simulink model "gm_HDL_pfc_gold_fi_og"  (R2024b)
settings: Solver=FixedStepDiscrete  StartTime=0.0  StopTime=.2  RelTol=1e-3
InitFcn:
  | fidelity_pfc_vals;
  | nbits=(2^12)-2;
  | A_mat = fi(stateSpaceParameters_1.Ad,1,25,24);
  | B_mat = fi(stateSpaceParameters_1.Bd,1,25,31);
  | C_mat = fi(stateSpaceParameters_1.Cd,1,25,20);
  | D_mat = fi(stateSpaceParameters_1.Dd,1,25,19);
  | X0_mat= fi(stateSpaceParameters_1.X0,1,25,14);
  | load('C:\Users\Angel\Desktop\hil\pfc3ph\matlab\sim\sschdl\pfc_desktop\stateSpaceParameters.mat');
undefined symbols (not defined in the file or in its folder): a, b, c, fsw, t_ss, tsw
libraries: simulink x39, hdlmdlgenlib x24, hdlsllib x9, mcbcontrolslib x5, dspsrcs4 x3, slpidlib x2, spsSVPWMGenerator2LevelLib x1, spsPLL3phLib x1, fillib x1
(part 1 of 4)
settings Model: Creator=angro  LastModifiedBy=Angel
settings OptimizationCC: BlockReduction=off  ConditionallyExecuteInputs=off  DefaultParameterBehavior=Inlined  InheritOutputTypeSmallerThanSingle=on  DefaultUnderspecifiedDataType=single
settings DebuggingCC: SignalRangeChecking=warning  AlgebraicLoopMsg=none  ArtificialAlgebraicLoopMsg=error  InheritedTsInSrcMsg=none  SingleTaskRateTransMsg=error  UnconnectedInputMsg=warning  UnconnectedOutputMsg=warning  UnconnectedLineMsg=warning
settings HardwareCC: ProdBitPerPointer=32  ProdBitPerSizeT=32  ProdBitPerPtrDiffT=32  ProdLargestAtomicFloat=None  ProdIntDivRoundTo=Undefined  ProdEndianess=Unspecified  ProdWordSize=32  ProdHWDeviceType=ASIC/FPGA->ASIC/FPGA  TargetBitPerPointer=64  TargetBitPerSizeT=64  TargetBitPerPtrDiffT=64  TargetLongLongMode=on  TargetIntDivRoundTo=Zero  TargetEndianess=LittleEndian  TargetWordSize=64  TargetHWDeviceType=Custom Processor->MATLAB Host Computer  ProdEqTarget=off

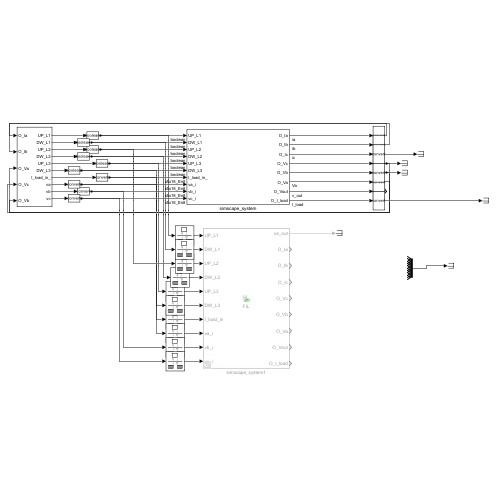
[thumbnail: Simulink's stored preview of the top-level diagram]
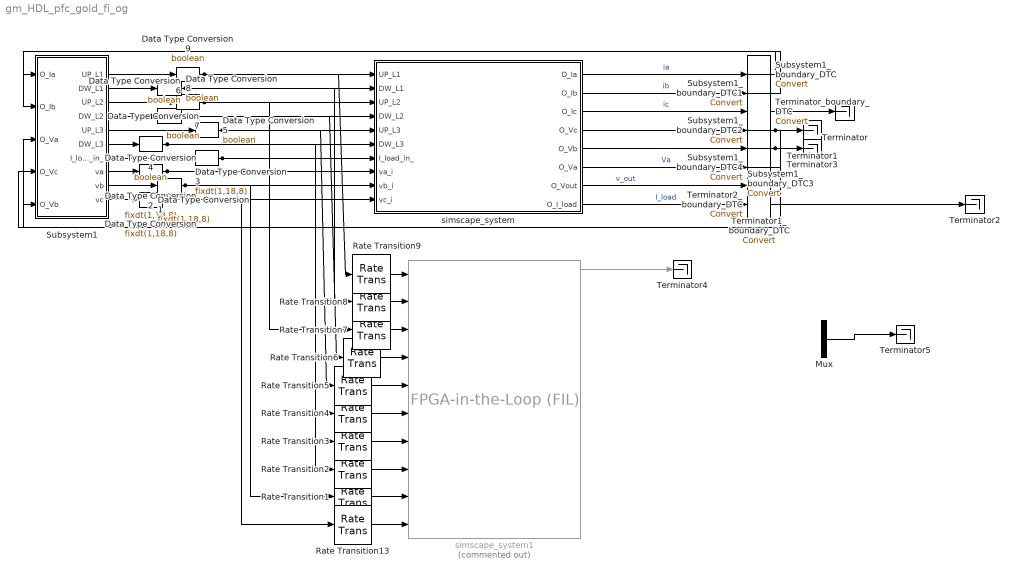
== system gm_HDL_pfc_gold_fi_og ==
  Data Type Conversion{,1..3} (4 alike) : DataTypeConversion  OutDataTypeStr=fixdt(1,18,8)  SaturateOnIntegerOverflow=off  RndMeth=Floor
  Data Type Conversion{4..9} (6 alike) : DataTypeConversion  OutDataTypeStr=boolean  SaturateOnIntegerOverflow=off  RndMeth=Floor
  Mux : Mux  Inputs=9
  Rate Transition{1..9,13} (10 alike) : RateTransition
  Subsystem1 : Subsystem
  Subsystem1_boundary_DTC{,1..4} (5 alike) : DataTypeConversion
  Terminator{,1..5} (6 alike) : Terminator
  Terminator1_boundary_DTC : DataTypeConversion
  Terminator2_boundary_DTC : DataTypeConversion
  Terminator_boundary_DTC : DataTypeConversion
  simscape_system : Subsystem
  simscape_system1 : fillib/FPGA-in-the-Loop (FIL)  Commented=on  ForceInterfaceUpdate=0.63368
  wires:
  simscape_system/8(O_I_load) -> Terminator2_boundary_DTC/1  "I_load"
  simscape_system/7(O_Vout) -> Terminator1_boundary_DTC/1  "v_out"
  simscape_system/6(O_Va) -> Subsystem1_boundary_DTC4/1  "Va"
  simscape_system/5(O_Vb) -> Subsystem1_boundary_DTC3/1
  simscape_system/4(O_Vc) -> Subsystem1_boundary_DTC2/1
  simscape_system/3(O_Ic) -> Terminator_boundary_DTC/1  "ic"
  simscape_system/2(O_Ib) -> Subsystem1_boundary_DTC1/1  "ib"
  simscape_system/1(O_Ia) -> Subsystem1_boundary_DTC/1  "ia"
  Mux/1 -> Terminator5/1
  Rate Transition9/1 -> simscape_system1/1
  Rate Transition8/1 -> simscape_system1/2
  Rate Transition7/1 -> simscape_system1/3
  Rate Transition6/1 -> simscape_system1/4
  Rate Transition5/1 -> simscape_system1/5
  Rate Transition4/1 -> simscape_system1/6
  Rate Transition3/1 -> simscape_system1/7
  Rate Transition2/1 -> simscape_system1/8
  Rate Transition1/1 -> simscape_system1/9
  Rate Transition13/1 -> simscape_system1/10
  simscape_system1/1 -> Terminator4/1
  Subsystem1_boundary_DTC4/1 -> Subsystem1/3(O_Va)
  Subsystem1_boundary_DTC3/1 -> Subsystem1/5(O_Vb), Terminator3/1
  Subsystem1_boundary_DTC2/1 -> Subsystem1/4(O_Vc), Terminator1/1
  Subsystem1_boundary_DTC1/1 -> Subsystem1/2(O_Ib)
  Subsystem1_boundary_DTC/1 -> Subsystem1/1(O_Ia)
  Terminator2_boundary_DTC/1 -> Terminator2/1
  Terminator_boundary_DTC/1 -> Terminator/1
  Data Type Conversion9/1 -> Rate Transition9/1, simscape_system/1(UP_L1)
  Data Type Conversion8/1 -> Rate Transition8/1, simscape_system/2(DW_L1)
  Data Type Conversion7/1 -> simscape_system/3(UP_L2), Rate Transition7/1
  Data Type Conversion6/1 -> Rate Transition6/1, simscape_system/4(DW_L2)
  Data Type Conversion5/1 -> Rate Transition5/1, simscape_system/5(UP_L3)
  Data Type Conversion4/1 -> Rate Transition4/1, simscape_system/6(DW_L3)
  Data Type Conversion3/1 -> Rate Transition3/1, simscape_system/7(I_load_in_)
  Data Type Conversion2/1 -> Rate Transition2/1, simscape_system/8(va_i)
  Data Type Conversion1/1 -> simscape_system/9(vb_i), Rate Transition1/1
  Data Type Conversion/1 -> simscape_system/10(vc_i), Rate Transition13/1
  Subsystem1/10(vc) -> Data Type Conversion/1
  Subsystem1/9(vb) -> Data Type Conversion1/1
  Subsystem1/8(va) -> Data Type Conversion2/1
  Subsystem1/6(DW_L3) -> Data Type Conversion4/1
  Subsystem1/5(UP_L3) -> Data Type Conversion5/1
  Subsystem1/4(DW_L2) -> Data Type Conversion6/1
  Subsystem1/3(UP_L2) -> Data Type Conversion7/1
  Subsystem1/2(DW_L1) -> Data Type Conversion8/1
  Subsystem1/1(UP_L1) -> Data Type Conversion9/1
  Subsystem1/7(I_load_in_) -> Data Type Conversion3/1

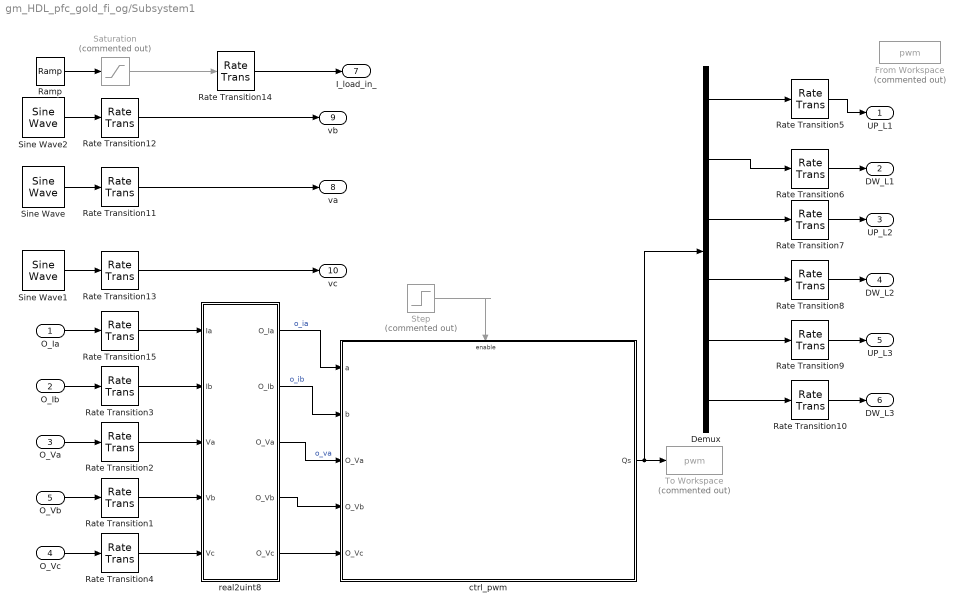
== system gm_HDL_pfc_gold_fi_og/Subsystem1 ==
  O_Ia : Inport
  O_Ib : Inport  Port=2
  O_Va : Inport  Port=3
  O_Vc : Inport  Port=4
  O_Vb : Inport  Port=5
  Demux : Demux  Outputs=6
  From Workspace : FromWorkspace  Commented=on  VariableName=pwm  SampleTime=t_ss  Interpolate=off  ZeroCross=off  OutputAfterFinalValue=Holding final value
  Ramp : simulink/Sources/Ramp  slope=1/50  start=2/50  InitialOutput=0
  Rate Transition{1..13,15} (14 alike) : RateTransition
  Rate Transition14 : RateTransition  OutPortSampleTime=t_ss
  Saturation : Saturate  Commented=on  UpperLimit=2
  Sine Wave : dspsrcs4/Sine Wave  Amplitude=325  Frequency=50  Phase=0  SampleMode=Discrete  OutComplex=Real  CompMethod=Table lookup  TableSize=Speed  SampleTime=tsw  SamplesPerFrame=1  ResetState=Restart at time zero  OutputFrames=off  dataType=double  wordLen=16  udDataType=sfix(16)  fracBitsMode=Best precision  numFracBits=15  OutDataTypeStr=double  LastOutDataTypeStr=double
  Sine Wave1 : dspsrcs4/Sine Wave  Amplitude=325  Frequency=50  Phase=2*pi/3  SampleMode=Discrete  OutComplex=Real  CompMethod=Table lookup  TableSize=Speed  SampleTime=tsw  SamplesPerFrame=1  ResetState=Restart at time zero  OutputFrames=off  dataType=double  wordLen=16  udDataType=sfix(16)  fracBitsMode=Best precision  numFracBits=15  OutDataTypeStr=double  LastOutDataTypeStr=double
  Sine Wave2 : dspsrcs4/Sine Wave  Amplitude=325  Frequency=50  Phase=-2*pi/3  SampleMode=Discrete  OutComplex=Real  CompMethod=Table lookup  TableSize=Speed  SampleTime=tsw  SamplesPerFrame=1  ResetState=Restart at time zero  OutputFrames=off  dataType=double  wordLen=16  udDataType=sfix(16)  fracBitsMode=Best precision  numFracBits=15  OutDataTypeStr=double  LastOutDataTypeStr=double
  Step : Step  Commented=on  Time=2/50  SampleTime=0
  To Workspace : ToWorkspace  Commented=on  VariableName=pwm  SaveFormat=Timeseries  SampleTime=-1
  ctrl_pwm : Subsystem
  real2uint8 : Subsystem
  UP_L1 : Outport
  DW_L1 : Outport  Port=2
  UP_L2 : Outport  Port=3
  DW_L2 : Outport  Port=4
  UP_L3 : Outport  Port=5
  DW_L3 : Outport  Port=6
  I_load_in_ : Outport  Port=7
  va : Outport  Port=8
  vb : Outport  Port=9
  vc : Outport  Port=10
  wires:
  Rate Transition9/1 -> UP_L3/1
  Rate Transition7/1 -> UP_L2/1
  Rate Transition6/1 -> DW_L1/1
  Rate Transition5/1 -> UP_L1/1
  Demux/4 -> Rate Transition8/1
  Demux/3 -> Rate Transition7/1
  Demux/2 -> Rate Transition6/1
  Demux/6 -> Rate Transition10/1
  Demux/1 -> Rate Transition5/1
  Demux/5 -> Rate Transition9/1
  ctrl_pwm/1(Qs) -> To Workspace/1, Demux/1
  real2uint8/5(O_Vc) -> ctrl_pwm/5(O_Vc)
  real2uint8/3(O_Va) -> ctrl_pwm/3(O_Va)  "o_va"
  real2uint8/2(O_Ib) -> ctrl_pwm/2(b)  "o_ib"
  real2uint8/1(O_Ia) -> ctrl_pwm/1(a)  "o_ia"
  real2uint8/4(O_Vb) -> ctrl_pwm/4(O_Vb)
  Step/1 -> ctrl_pwm/Enable
  Rate Transition14/1 -> I_load_in_/1
  Rate Transition10/1 -> DW_L3/1
  Rate Transition4/1 -> real2uint8/5(Vc)
  Rate Transition13/1 -> vc/1
  Rate Transition1/1 -> real2uint8/4(Vb)
  Rate Transition11/1 -> va/1
  Rate Transition3/1 -> real2uint8/2(Ib)
  Rate Transition12/1 -> vb/1
  Rate Transition2/1 -> real2uint8/3(Va)
  O_Vc/1 -> Rate Transition4/1
  O_Ia/1 -> Rate Transition15/1
  O_Va/1 -> Rate Transition2/1
  O_Vb/1 -> Rate Transition1/1
  O_Ib/1 -> Rate Transition3/1
  Sine Wave/1 -> Rate Transition11/1
  Rate Transition8/1 -> DW_L2/1
  Sine Wave1/1 -> Rate Transition13/1
  Saturation/1 -> Rate Transition14/1
  Sine Wave2/1 -> Rate Transition12/1
  Rate Transition15/1 -> real2uint8/1(Ia)
  Ramp/1 -> Saturation/1

== system gm_HDL_pfc_gold_fi_og/simscape_system ==
  UP_L1 : Inport  OutDataTypeStr=boolean  PortDimensions=1  SampleTime=5.12820512820513e-07
  DW_L1 : Inport  Port=2  OutDataTypeStr=boolean  PortDimensions=1  SampleTime=5.12820512820513e-07
  UP_L2 : Inport  Port=3  OutDataTypeStr=boolean  PortDimensions=1  SampleTime=5.12820512820513e-07
  DW_L2 : Inport  Port=4  OutDataTypeStr=boolean  PortDimensions=1  SampleTime=5.12820512820513e-07
  UP_L3 : Inport  Port=5  OutDataTypeStr=boolean  PortDimensions=1  SampleTime=5.12820512820513e-07
  DW_L3 : Inport  Port=6  OutDataTypeStr=boolean  PortDimensions=1  SampleTime=5.12820512820513e-07
  I_load_in_ : Inport  Port=7  OutDataTypeStr=fixdt(1, 18, 8)  PortDimensions=1  SampleTime=5.12820512820513e-07
  va_i : Inport  Port=8  OutDataTypeStr=fixdt(1, 18, 8)  PortDimensions=1  SampleTime=5.12820512820513e-07  LockScale=on
  vb_i : Inport  Port=9  OutDataTypeStr=fixdt(1, 18, 8)  PortDimensions=1  SampleTime=5.12820512820513e-07  LockScale=on
  vc_i : Inport  Port=10  OutDataTypeStr=fixdt(1, 18, 8)  PortDimensions=1  SampleTime=5.12820512820513e-07  LockScale=on
  simscape_system : Subsystem
  t{,1..7} (8 alike) : RateTransition  InitialCondition=double(0)  OutPortSampleTimeOpt=Multiple of input port sample time  OutPortSampleTimeMultiple=49
  O_Ia : Outport  SampleTime=5.12820512820513e-07
  O_Ib : Outport  Port=2  SampleTime=5.12820512820513e-07
  O_Ic : Outport  Port=3  SampleTime=5.12820512820513e-07
  O_Vc : Outport  Port=4  SampleTime=5.12820512820513e-07
  O_Vb : Outport  Port=5  SampleTime=5.12820512820513e-07
  O_Va : Outport  Port=6  SampleTime=5.12820512820513e-07
  O_Vout : Outport  Port=7  SampleTime=5.12820512820513e-07
  O_I_load : Outport  Port=8  SampleTime=5.12820512820513e-07
  wires:
  UP_L1/1 -> simscape_system/1(UP_L1)
  DW_L1/1 -> simscape_system/2(DW_L1)
  UP_L3/1 -> simscape_system/5(UP_L3)
  UP_L2/1 -> simscape_system/3(UP_L2)
  DW_L2/1 -> simscape_system/4(DW_L2)
  I_load_in_/1 -> simscape_system/7(I_load_in_)
  DW_L3/1 -> simscape_system/6(DW_L3)
  va_i/1 -> simscape_system/8(va_i)
  vb_i/1 -> simscape_system/9(vb_i)
  vc_i/1 -> simscape_system/10(vc_i)
  t1/1 -> O_Ic/1
  simscape_system/1(O_Ia) -> t7/1
  simscape_system/2(O_Ib) -> t/1
  simscape_system/3(O_Ic) -> t1/1
  simscape_system/4(O_Vc) -> t2/1
  simscape_system/5(O_Vb) -> t3/1
  simscape_system/6(O_Va) -> t4/1
  t6/1 -> O_I_load/1
  simscape_system/7(O_Vout) -> t5/1
  simscape_system/8(O_I_load) -> t6/1
  t7/1 -> O_Ia/1
  t/1 -> O_Ib/1
  t2/1 -> O_Vc/1
  t3/1 -> O_Vb/1
  t4/1 -> O_Va/1
  t5/1 -> O_Vout/1

== system gm_HDL_pfc_gold_fi_og/Subsystem1/ctrl_pwm ==
  a : Inport
  b : Inport  Port=2
  O_Va : Inport  Port=3
  O_Vb : Inport  Port=4
  O_Vc : Inport  Port=5
  Enable : EnablePort
  PI_CTRL : Subsystem
  SVPWM : Subsystem
  transforms : Subsystem
  Qs : Outport
  wires:
  O_Vb/1 -> transforms/4(In4)
  O_Va/1 -> transforms/3(In3)
  b/1 -> transforms/2(b)
  PI_CTRL/2(Vq_inductor) -> SVPWM/3(Vq_inductor)
  SVPWM/1(P) -> Qs/1  "Qs"
  transforms/2(iq) -> PI_CTRL/2(iq)
  O_Vc/1 -> transforms/5(In5)
  a/1 -> transforms/1(a)
  PI_CTRL/1(Vd_inductor) -> SVPWM/1(Vd_inductor)
  transforms/3(angle) -> SVPWM/2(angle)
  transforms/1(id) -> PI_CTRL/1(id)

== system gm_HDL_pfc_gold_fi_og/Subsystem1/real2uint8 ==
  Ia : Inport
  Ib : Inport  Port=2
  Va : Inport  Port=3
  Vb : Inport  Port=4
  Vc : Inport  Port=5
  Add2 : Sum  Inputs=-+  OutDataTypeStr=Inherit: Same as first input
  Add3 : Sum  Inputs=+-
  Constant : Constant  Value=40  SampleTime=-1
  Constant1 : Constant  Value=420  SampleTime=-1
  Demux : Demux  Outputs=3
  Demux1 : Demux  Outputs=2
  Gain2 : Gain  Gain=80/nbits  OutDataTypeStr=Inherit: Same as input
  Gain5 : Gain  Gain=840/nbits  OutDataTypeStr=Inherit: Same as input
  Mux : Mux  Inputs=3
  Mux1 : Mux  Inputs=2
  O_Ia : Outport
  O_Ib : Outport  Port=2
  O_Va : Outport  Port=3
  O_Vb : Outport  Port=4
  O_Vc : Outport  Port=5
  wires:
  Add3/1 -> Demux/1
  Add2/1 -> Demux1/1
  Gain2/1 -> Add2/2
  Gain5/1 -> Add3/1
  Mux/1 -> Gain5/1
  Mux1/1 -> Gain2/1
  Demux1/2 -> O_Ia/1
  Demux1/1 -> O_Ib/1
  Demux/3 -> O_Va/1
  Demux/2 -> O_Vc/1
  Constant/1 -> Add2/1
  Constant1/1 -> Add3/2
  Demux/1 -> O_Vb/1
  Ib/1 -> Mux1/1
  Vc/1 -> Mux/2
  Ia/1 -> Mux1/2  "rIA"
  Vb/1 -> Mux/1
  Va/1 -> Mux/3

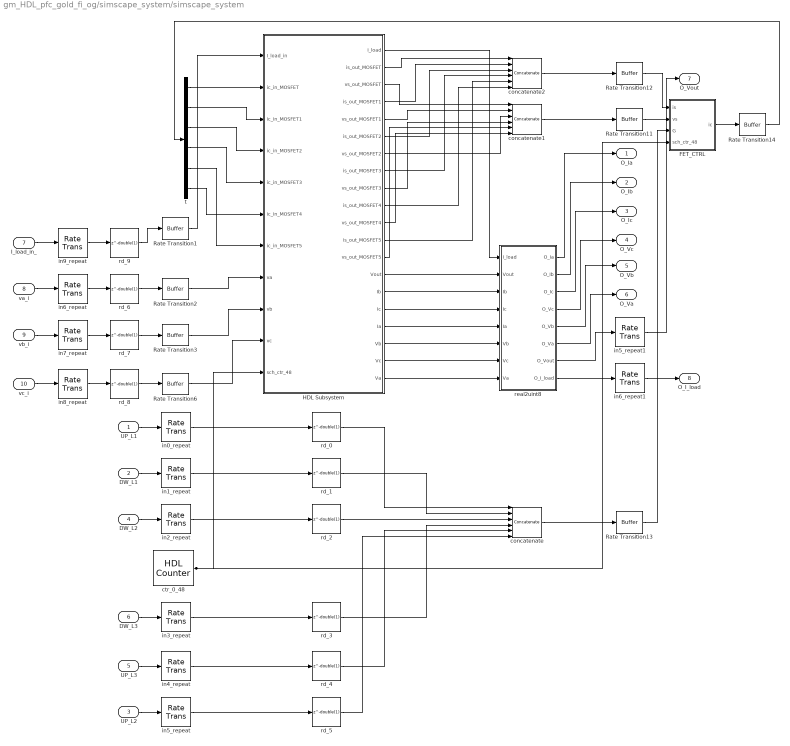
== system gm_HDL_pfc_gold_fi_og/simscape_system/simscape_system ==
  UP_L1 : Inport  OutDataTypeStr=boolean  SampleTime=5.12820512820513e-07
  DW_L1 : Inport  Port=2  OutDataTypeStr=boolean  SampleTime=5.12820512820513e-07
  UP_L2 : Inport  Port=3  OutDataTypeStr=boolean  SampleTime=5.12820512820513e-07
  DW_L2 : Inport  Port=4  OutDataTypeStr=boolean  SampleTime=5.12820512820513e-07
  UP_L3 : Inport  Port=5  OutDataTypeStr=boolean  SampleTime=5.12820512820513e-07
  DW_L3 : Inport  Port=6  OutDataTypeStr=boolean  SampleTime=5.12820512820513e-07
  I_load_in_ : Inport  Port=7  OutDataTypeStr=fixdt(1, 18, 8)  SampleTime=5.12820512820513e-07
  va_i : Inport  Port=8  OutDataTypeStr=fixdt(1, 18, 8)  SampleTime=5.12820512820513e-07
  vb_i : Inport  Port=9  OutDataTypeStr=fixdt(1, 18, 8)  SampleTime=5.12820512820513e-07
  vc_i : Inport  Port=10  OutDataTypeStr=fixdt(1, 18, 8)  SampleTime=5.12820512820513e-07
  FET_CTRL : Subsystem
  HDL Subsystem : Subsystem
  Rate Transition{1..3,6,11..14} (8 alike) : hdlmdlgenlib/Buffer
  concatenate : Concatenate  NumInputs=6
  concatenate1 : Concatenate  NumInputs=6
  concatenate2 : Concatenate  NumInputs=6
  ctr_0_48 : hdlsllib/Sources/HDL Counter  CountType=Count limited  CountInit=double(0)  CountStep=double(1)  CountMax=double(48)  CountFromType=Initial value  CountFrom=double(0)  CountResetPort=off  CountLoadPort=off  CountEnbPort=off  CountDirPort=off  CountHitOutputPort=off  CountDataType=Unsigned  CountWordLen=6  CountFracLen=0  CountSampTime=1.0465724751439e-08
  in0_repeat : RateTransition  Integrity=off  Deterministic=off  OutPortSampleTimeOpt=Multiple of input port sample time  OutPortSampleTimeMultiple=1/49
  in1_repeat : RateTransition  Integrity=off  Deterministic=off  OutPortSampleTimeOpt=Multiple of input port sample time  OutPortSampleTimeMultiple=1/49
  in2_repeat : RateTransition  Integrity=off  Deterministic=off  OutPortSampleTimeOpt=Multiple of input port sample time  OutPortSampleTimeMultiple=1/49
  in3_repeat : RateTransition  Integrity=off  Deterministic=off  OutPortSampleTimeOpt=Multiple of input port sample time  OutPortSampleTimeMultiple=1/49
  in4_repeat : RateTransition  Integrity=off  Deterministic=off  OutPortSampleTimeOpt=Multiple of input port sample time  OutPortSampleTimeMultiple=1/49
  in5_repeat : RateTransition  Integrity=off  Deterministic=off  OutPortSampleTimeOpt=Multiple of input port sample time  OutPortSampleTimeMultiple=1/49
  in5_repeat1 : RateTransition  Integrity=off  Deterministic=off  OutPortSampleTimeOpt=Multiple of input port sample time  OutPortSampleTimeMultiple=1/49
  in6_repeat : RateTransition  Integrity=off  Deterministic=off  OutPortSampleTimeOpt=Multiple of input port sample time  OutPortSampleTimeMultiple=1/49
  in6_repeat1 : RateTransition  Integrity=off  Deterministic=off  OutPortSampleTimeOpt=Multiple of input port sample time  OutPortSampleTimeMultiple=1/49
  in7_repeat : RateTransition  Integrity=off  Deterministic=off  OutPortSampleTimeOpt=Multiple of input port sample time  OutPortSampleTimeMultiple=1/49
  in8_repeat : RateTransition  Integrity=off  Deterministic=off  OutPortSampleTimeOpt=Multiple of input port sample time  OutPortSampleTimeMultiple=1/49
  in9_repeat : RateTransition  Integrity=off  Deterministic=off  OutPortSampleTimeOpt=Multiple of input port sample time  OutPortSampleTimeMultiple=1/49
  rd_{0..9} (10 alike) : Delay  DelayLength=double(1)  InitialCondition=0  SampleTime=1.0465724751439e-08
  real2uint8 : Subsystem
  t : Demux  Outputs=6
  O_Ia : Outport  OutDataTypeStr=uint16  SampleTime=1.0465724751439e-08
  O_Ib : Outport  Port=2  OutDataTypeStr=uint16  SampleTime=1.0465724751439e-08
  O_Ic : Outport  Port=3  OutDataTypeStr=uint16  SampleTime=1.0465724751439e-08
  O_Vc : Outport  Port=4  OutDataTypeStr=uint16  SampleTime=1.0465724751439e-08
  O_Vb : Outport  Port=5  OutDataTypeStr=uint16  SampleTime=1.0465724751439e-08
  O_Va : Outport  Port=6  OutDataTypeStr=uint16  SampleTime=1.0465724751439e-08
  O_Vout : Outport  Port=7  OutDataTypeStr=uint16  SampleTime=1.0465724751439e-08
  O_I_load : Outport  Port=8  OutDataTypeStr=uint16  SampleTime=1.0465724751439e-08
  wires:
  DW_L3/1 -> in3_repeat/1
  I_load_in_/1 -> in9_repeat/1
  va_i/1 -> in6_repeat/1
  in6_repeat/1 -> rd_6/1
  vb_i/1 -> in7_repeat/1
  in2_repeat/1 -> rd_2/1
  DW_L1/1 -> in1_repeat/1
  vc_i/1 -> in8_repeat/1
  in9_repeat/1 -> rd_9/1
  Rate Transition1/1 -> HDL Subsystem/1(I_load_in)
  HDL Subsystem/12(is_out_MOSFET5) -> concatenate2/5
  HDL Subsystem/2(is_out_MOSFET) -> concatenate2/1
  Rate Transition14/1 -> t/1
  in3_repeat/1 -> rd_3/1
  in7_repeat/1 -> rd_7/1
  real2uint8/1(O_Ia) -> O_Ia/1
  rd_1/1 -> concatenate/2
  rd_8/1 -> Rate Transition6/1
  in8_repeat/1 -> rd_8/1
  rd_9/1 -> Rate Transition1/1
  Rate Transition6/1 -> HDL Subsystem/10(vc)
  rd_6/1 -> Rate Transition2/1
  rd_7/1 -> Rate Transition3/1
  HDL Subsystem/1(I_load) -> real2uint8/1(I_load)
  in0_repeat/1 -> rd_0/1
  UP_L1/1 -> in0_repeat/1
  DW_L2/1 -> in2_repeat/1
  UP_L3/1 -> in4_repeat/1
  HDL Subsystem/6(is_out_MOSFET2) -> concatenate2/3
  in4_repeat/1 -> rd_4/1
  ctr_0_48/1 -> FET_CTRL/4(sch_ctr_48), HDL Subsystem/11(sch_ctr_48)
  UP_L2/1 -> in5_repeat/1
  t/1 -> HDL Subsystem/2(ic_in_MOSFET)
  HDL Subsystem/19(Vc) -> real2uint8/7(Vc)
  t/2 -> HDL Subsystem/3(ic_in_MOSFET1)
  HDL Subsystem/18(Vb) -> real2uint8/6(Vb)
  t/3 -> HDL Subsystem/4(ic_in_MOSFET2)
  t/4 -> HDL Subsystem/5(ic_in_MOSFET3)
  Rate Transition11/1 -> FET_CTRL/2(vs)
  t/6 -> HDL Subsystem/6(ic_in_MOSFET4)
  t/5 -> HDL Subsystem/7(ic_in_MOSFET5)
  HDL Subsystem/13(vs_out_MOSFET5) -> concatenate1/5
  HDL Subsystem/4(is_out_MOSFET1) -> concatenate2/2
  Rate Transition2/1 -> HDL Subsystem/8(va)
  Rate Transition3/1 -> HDL Subsystem/9(vb)
  HDL Subsystem/20(Va) -> real2uint8/8(Va)
  in1_repeat/1 -> rd_1/1
  HDL Subsystem/17(Ia) -> real2uint8/5(Ia)
  in5_repeat/1 -> rd_5/1
  HDL Subsystem/3(vs_out_MOSFET) -> concatenate1/1
  HDL Subsystem/5(vs_out_MOSFET1) -> concatenate1/2
  HDL Subsystem/7(vs_out_MOSFET2) -> concatenate1/3
  HDL Subsystem/8(is_out_MOSFET3) -> concatenate2/4
  HDL Subsystem/9(vs_out_MOSFET3) -> concatenate1/4
  HDL Subsystem/10(is_out_MOSFET4) -> concatenate2/6
  HDL Subsystem/11(vs_out_MOSFET4) -> concatenate1/6
  HDL Subsystem/14(Vout) -> real2uint8/2(Vout)
  HDL Subsystem/15(Ib) -> real2uint8/3(Ib)
  HDL Subsystem/16(Ic) -> real2uint8/4(Ic)
  rd_0/1 -> concatenate/1
  rd_2/1 -> concatenate/3
  rd_3/1 -> concatenate/4
  rd_4/1 -> concatenate/5
  concatenate1/1 -> Rate Transition11/1
  rd_5/1 -> concatenate/6
  concatenate2/1 -> Rate Transition12/1
  real2uint8/2(O_Ib) -> O_Ib/1
  real2uint8/3(O_Ic) -> O_Ic/1
  real2uint8/4(O_Vc) -> O_Vc/1
  real2uint8/5(O_Vb) -> O_Vb/1
  real2uint8/6(O_Va) -> O_Va/1
  real2uint8/7(O_Vout) -> in5_repeat1/1
  real2uint8/8(O_I_load) -> in6_repeat1/1
  concatenate/1 -> Rate Transition13/1
  Rate Transition12/1 -> FET_CTRL/1(is)
  in5_repeat1/1 -> O_Vout/1
  in6_repeat1/1 -> O_I_load/1
  Rate Transition13/1 -> FET_CTRL/3(G)
  FET_CTRL/1(ic) -> Rate Transition14/1

== system gm_HDL_pfc_gold_fi_og/Subsystem1/ctrl_pwm/PI_CTRL ==
  id : Inport
  iq : Inport  Port=2
  Add3 : Sum  Inputs=+-
  Add4 : Sum  Inputs=+-
  Constant : Constant  Value=0  SampleTime=t_ss
  Constant1 : Constant  Value=-4  SampleTime=t_ss
  Vd_ctrl : slpidlib/PID Controller  Controller=PI  Form=Parallel  TimeDomain=Discrete-time  UseExternalTs=off  SampleTime=-1  IntegratorMethod=Backward Euler  FilterMethod=Forward Euler  ControllerParametersSource=internal  P=-1.8  I=-.15  UseKiTs=off  D=0  UseExternalDerivativeSource=off  N=100  UseFilter=on  TunerSelectOption=Transfer Function Based (PID Tuner App)  InitialConditionSource=internal  InitialConditionForIntegrator=0  InitialConditionForFilter=0  DifferentiatorICPrevScaledInput=0  ExternalReset=none  TrackingMode=off  Kt=1  LimitOutput=off  SatLimitsSource=internal  UpperSaturationLimit=5e2  LowerSaturationLimit=-5e2  LinearizeAsGain=on  AntiWindupMode=clamping  Kb=1  LimitIntegrator=off  UpperIntegratorSaturationLimit=inf  LowerIntegratorSaturationLimit=-inf  POutMin=[]  POutMax=[]  IOutMin=[]  IOutMax=[]  DOutMin=[]  DOutMax=[]  NOutMin=[]  NOutMax=[]  SumOutMin=[]  SumOutMax=[]  SaturationOutMin=[]  SaturationOutMax=[]  PParamMin=[]  PParamMax=[]  IParamMin=[]  IParamMax=[]  DParamMin=[]  DParamMax=[]  NParamMin=[]  NParamMax=[]  KbParamMin=[]  KbParamMax=[]  KtParamMin=[]  KtParamMax=[]  KbOutMin=[]  KbOutMax=[]  KtOutMin=[]  KtOutMax=[]  IntegratorOutMin=[]  IntegratorOutMax=[]  FilterOutMin=[]  FilterOutMax=[]  SumI1OutMin=[]  SumI1OutMax=[]  SumI2OutMin=[]  SumI2OutMax=[]  SumI3OutMin=[]  SumI3OutMax=[]  SumI4OutMin=[]  SumI4OutMax=[]  SumDOutMin=[]  SumDOutMax=[]  DifferentiatorOutMin=[]  DifferentiatorOutMax=[]  FilterDiffOutCoefMin=[]  FilterDiffOutCoefMax=[]  ReciprocalOutMin=[]  ReciprocalOutMax=[]  SumDenOutMin=[]  SumDenOutMax=[]  SumNumOutMin=[]  SumNumOutMax=[]  DivideOutMin=[]  DivideOutMax=[]  UdiffTsProdOutMin=[]  UdiffTsProdOutMax=[]  NTsProdOutMin=[]  NTsProdOutMax=[]  UintegralTsProdOutMin=[]  UintegralTsProdOutMax=[]  UngainTsProdOutMin=[]  UngainTsProdOutMax=[]  ClampingZeroOutDataTypeStr=Inherit: Inherit via back propagation  ClampingZeroOutMin=[]  ClampingZeroOutMax=[]  FilterDenConstantOutDataTypeStr=Inherit: Inherit via back propagation  FilterDenConstantOutMin=[]  FilterDenConstantOutMax=[]  PCopyOutDataTypeStr=Inherit: Inherit via back propagation  PCopyOutMin=[]  PCopyOutMax=[]  NCopyOutDataTypeStr=Inherit: Inherit via back propagation  NCopyOutMin=[]  NCopyOutMax=[]  IntegratorContinuousStateAttributes=''  IntegratorStateMustResolveToSignalObject=off  IntegratorRTWStateStorageClass=Auto  FilterContinuousStateAttributes=''  FilterStateMustResolveToSignalObject=off  FilterRTWStateStorageClass=Auto  ParallelPVariant=InternalParameters  IdealPVariant=Disabled  IVariant=InternalParameters  DVariant=Disabled  IntegratorVariant=Discrete  SatVariant=Disabled  AWVariant=Passthrough  PCopyVariant=Disabled  TRVariant=Disabled  FdbkBlocksVariant=Forward  IdealPFdbkVariant=Disabled  SatFdbkVariant=Disabled  DerivativeFilterVariant=Disabled  NVariant=Disabled  NCopyVariant=Disabled_SignalSpec  FilterICVariant=Disabled  IntegratorICVariant=InternalICs  ExternalResetVariant=Disabled  TRSumVariant=Passthrough  SumFdbkVariant=Disabled  SumVariant=Sum_PI  TsampFilterVariant=InternalTs  TsampNgainVariant=Passthrough  TsampIntegralVariant=Disabled_SignalSpec  ExternalSaturationOutDataTypeStr=Inherit: Same as second input  DerivativeSourceVariant=Disabled  PreIntVariant=InternalPreInt
  Vq_ctrl : slpidlib/PID Controller  Controller=PI  Form=Parallel  TimeDomain=Discrete-time  UseExternalTs=off  SampleTime=-1  IntegratorMethod=Backward Euler  FilterMethod=Forward Euler  ControllerParametersSource=internal  P=-2  I=-.2  UseKiTs=off  D=0  UseExternalDerivativeSource=off  N=100  UseFilter=on  TunerSelectOption=Transfer Function Based (PID Tuner App)  InitialConditionSource=internal  InitialConditionForIntegrator=0  InitialConditionForFilter=0  DifferentiatorICPrevScaledInput=0  ExternalReset=none  TrackingMode=off  Kt=1  LimitOutput=off  SatLimitsSource=internal  UpperSaturationLimit=5e2  LowerSaturationLimit=-5e2  LinearizeAsGain=on  AntiWindupMode=clamping  Kb=1  LimitIntegrator=off  UpperIntegratorSaturationLimit=inf  LowerIntegratorSaturationLimit=-inf  POutMin=[]  POutMax=[]  IOutMin=[]  IOutMax=[]  DOutMin=[]  DOutMax=[]  NOutMin=[]  NOutMax=[]  SumOutMin=[]  SumOutMax=[]  SaturationOutMin=[]  SaturationOutMax=[]  PParamMin=[]  PParamMax=[]  IParamMin=[]  IParamMax=[]  DParamMin=[]  DParamMax=[]  NParamMin=[]  NParamMax=[]  KbParamMin=[]  KbParamMax=[]  KtParamMin=[]  KtParamMax=[]  KbOutMin=[]  KbOutMax=[]  KtOutMin=[]  KtOutMax=[]  IntegratorOutMin=[]  IntegratorOutMax=[]  FilterOutMin=[]  FilterOutMax=[]  SumI1OutMin=[]  SumI1OutMax=[]  SumI2OutMin=[]  SumI2OutMax=[]  SumI3OutMin=[]  SumI3OutMax=[]  SumI4OutMin=[]  SumI4OutMax=[]  SumDOutMin=[]  SumDOutMax=[]  DifferentiatorOutMin=[]  DifferentiatorOutMax=[]  FilterDiffOutCoefMin=[]  FilterDiffOutCoefMax=[]  ReciprocalOutMin=[]  ReciprocalOutMax=[]  SumDenOutMin=[]  SumDenOutMax=[]  SumNumOutMin=[]  SumNumOutMax=[]  DivideOutMin=[]  DivideOutMax=[]  UdiffTsProdOutMin=[]  UdiffTsProdOutMax=[]  NTsProdOutMin=[]  NTsProdOutMax=[]  UintegralTsProdOutMin=[]  UintegralTsProdOutMax=[]  UngainTsProdOutMin=[]  UngainTsProdOutMax=[]  ClampingZeroOutDataTypeStr=Inherit: Inherit via back propagation  ClampingZeroOutMin=[]  ClampingZeroOutMax=[]  FilterDenConstantOutDataTypeStr=Inherit: Inherit via back propagation  FilterDenConstantOutMin=[]  FilterDenConstantOutMax=[]  PCopyOutDataTypeStr=Inherit: Inherit via back propagation  PCopyOutMin=[]  PCopyOutMax=[]  NCopyOutDataTypeStr=Inherit: Inherit via back propagation  NCopyOutMin=[]  NCopyOutMax=[]  IntegratorContinuousStateAttributes=''  IntegratorStateMustResolveToSignalObject=off  IntegratorRTWStateStorageClass=Auto  FilterContinuousStateAttributes=''  FilterStateMustResolveToSignalObject=off  FilterRTWStateStorageClass=Auto  ParallelPVariant=InternalParameters  IdealPVariant=Disabled  IVariant=InternalParameters  DVariant=Disabled  IntegratorVariant=Discrete  SatVariant=Disabled  AWVariant=Passthrough  PCopyVariant=Disabled  TRVariant=Disabled  FdbkBlocksVariant=Forward  IdealPFdbkVariant=Disabled  SatFdbkVariant=Disabled  DerivativeFilterVariant=Disabled  NVariant=Disabled  NCopyVariant=Disabled_SignalSpec  FilterICVariant=Disabled  IntegratorICVariant=InternalICs  ExternalResetVariant=Disabled  TRSumVariant=Passthrough  SumFdbkVariant=Disabled  SumVariant=Sum_PI  TsampFilterVariant=InternalTs  TsampNgainVariant=Passthrough  TsampIntegralVariant=Disabled_SignalSpec  ExternalSaturationOutDataTypeStr=Inherit: Same as second input  DerivativeSourceVariant=Disabled  PreIntVariant=InternalPreInt
  Vd_inductor : Outport
  Vq_inductor : Outport  Port=2
  wires:
  Constant1/1 -> Add4/1
  Vq_ctrl/1 -> Vq_inductor/1
  Vd_ctrl/1 -> Vd_inductor/1
  Add4/1 -> Vq_ctrl/1  "error_iq"
  iq/1 -> Add4/2
  Constant/1 -> Add3/1
  id/1 -> Add3/2
  Add3/1 -> Vd_ctrl/1  "error_id"

== system gm_HDL_pfc_gold_fi_og/Subsystem1/ctrl_pwm/SVPWM ==
  Vd_inductor : Inport
  angle : Inport  Port=2
  Vq_inductor : Inport  Port=3
  Cos : Trigonometry  Operator=cos
  Inverse Park Transform : mcbcontrolslib/Inverse Park Transform  PhaseInput=Two inputs  AxisAlignment=D-axis  ThetaInput=Sine and Cosine electrical position  AngleInput=Per-unit  N_points=1024
  SVPWM Generator (2-Level) : spsSVPWMGenerator2LevelLib/SVPWM Generator (2-Level)  InputType=alpha-beta components  SwitchingPattern=Pattern #1  Fc=fsw*1e3  ParUref=[0.8 -30 50]  Ts=t_ss
  Sin : Trigonometry
  P : Outport
  wires:
  SVPWM Generator (2-Level)/1 -> P/1
  angle/1 -> Sin/1, Cos/1
  Inverse Park Transform/1 -> SVPWM Generator (2-Level)/1  "Valp_indc"
  Cos/1 -> Inverse Park Transform/4
  Sin/1 -> Inverse Park Transform/3
  Inverse Park Transform/2 -> SVPWM Generator (2-Level)/2  "Vbet_indc"
  Vq_inductor/1 -> Inverse Park Transform/2
  Vd_inductor/1 -> Inverse Park Transform/1

== system gm_HDL_pfc_gold_fi_og/Subsystem1/ctrl_pwm/transforms ==
  a : Inport
  b : Inport  Port=2
  In3 : Inport  Port=3
  In4 : Inport  Port=4
  In5 : Inport  Port=5
  Claro-Parl Transform : Subsystem  Commented=on
  Claro-Parl Transform1 : Subsystem
  Delay : Delay  DelayLength=1
  Delay1 : Delay  DelayLength=1
  Mux : Mux  Inputs=3
  PLL (3ph) : spsPLL3phLib/PLL (3ph)  Fmin=50  Par_Init=[0, 50]  ParK=[180,3200,1]  TcD=1e-4  MaxRateChangeFreq=12  FilterCutOffFreq=25  Ts=t_ss  AGC=on
  Terminator : Terminator
  id : Outport
  iq : Outport  Port=2
  angle : Outport  Port=3
  wires:
  Claro-Parl Transform1/2(q) -> iq/1  "iq"
  Claro-Parl Transform1/1(d) -> id/1  "id"
  Claro-Parl Transform/2(q) -> ?  "vq"
  Claro-Parl Transform/1(d) -> ?  "vd"
  Delay1/1 -> Claro-Parl Transform1/2(b)
  Delay/1 -> Claro-Parl Transform1/1(a)
  a/1 -> Delay/1
  In4/1 -> Mux/2, Claro-Parl Transform/2(b)
  b/1 -> Delay1/1
  In5/1 -> Mux/3
  In3/1 -> Claro-Parl Transform/1(a), Mux/1
  PLL (3ph)/1 -> Terminator/1
  PLL (3ph)/2 -> Claro-Parl Transform/3(wt), Claro-Parl Transform1/3(wt), angle/1  "angle"
  Mux/1 -> PLL (3ph)/1

== system gm_HDL_pfc_gold_fi_og/simscape_system/simscape_system/FET_CTRL ==
  is : Inport  OutDataTypeStr=fixdt(1, 18, 6)  PortDimensions=[6]  SampleTime=1.0465724751439e-08
  vs : Inport  Port=2  OutDataTypeStr=fixdt(1, 18, 6)  PortDimensions=[6]  SampleTime=1.0465724751439e-08
  G : Inport  Port=3  OutDataTypeStr=boolean  PortDimensions=[6]  SampleTime=1.0465724751439e-08
  sch_ctr_48 : Inport  Port=4  OutDataTypeStr=fixdt(0, 6, 0)  SampleTime=1.0465724751439e-08
  Discrete-Time Integrator_reg : RateTransition  InitialCondition=double(0)  OutPortSampleTimeOpt=Multiple of input port sample time  OutPortSampleTimeMultiple=49
  Discrete-Time Integrator_reg_absorbed : Delay  DelayLength=0
  crp_out_delay : Delay  DelayLength=double(1)  InitialCondition=0  SampleTime=1.0465724751439e-08
  crp_temp_streamed : Subsystem
  in0_repeat : RateTransition  Integrity=off  Deterministic=off  OutPortSampleTimeOpt=Multiple of input port sample time  OutPortSampleTimeMultiple=1/49
  ic : Outport  SampleTime=1.0465724751439e-08
  wires:
  crp_out_delay/1 -> Discrete-Time Integrator_reg/1
  in0_repeat/1 -> crp_temp_streamed/1(in0)
  G/1 -> crp_temp_streamed/2(in1)
  Discrete-Time Integrator_reg_absorbed/1 -> in0_repeat/1
  is/1 -> crp_temp_streamed/4(in3)
  vs/1 -> crp_temp_streamed/3(in2)
  crp_temp_streamed/1(out0) -> crp_out_delay/1
  sch_ctr_48/1 -> crp_temp_streamed/5(enb_counter)
  crp_temp_streamed/2(out1) -> ic/1
  Discrete-Time Integrator_reg/1 -> Discrete-Time Integrator_reg_absorbed/1

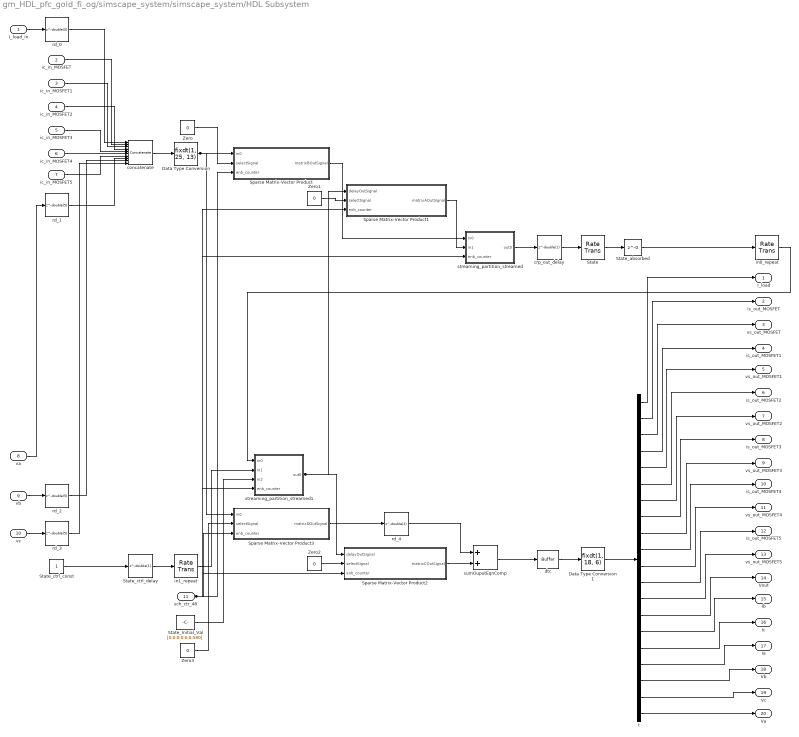
== system gm_HDL_pfc_gold_fi_og/simscape_system/simscape_system/HDL Subsystem ==
  I_load_in : Inport  OutDataTypeStr=fixdt(1, 18, 8)  PortDimensions=1  SampleTime=1.0465724751439e-08
  ic_in_MOSFET : Inport  Port=2  OutDataTypeStr=fixdt(1, 18, 8)  PortDimensions=1  SampleTime=1.0465724751439e-08
  ic_in_MOSFET1 : Inport  Port=3  OutDataTypeStr=fixdt(1, 18, 8)  PortDimensions=1  SampleTime=1.0465724751439e-08
  ic_in_MOSFET2 : Inport  Port=4  OutDataTypeStr=fixdt(1, 18, 8)  PortDimensions=1  SampleTime=1.0465724751439e-08
  ic_in_MOSFET3 : Inport  Port=5  OutDataTypeStr=fixdt(1, 18, 8)  PortDimensions=1  SampleTime=1.0465724751439e-08
  ic_in_MOSFET4 : Inport  Port=6  OutDataTypeStr=fixdt(1, 18, 8)  PortDimensions=1  SampleTime=1.0465724751439e-08
  ic_in_MOSFET5 : Inport  Port=7  OutDataTypeStr=fixdt(1, 18, 8)  PortDimensions=1  SampleTime=1.0465724751439e-08
  va : Inport  Port=8  OutDataTypeStr=fixdt(1, 18, 8)  PortDimensions=1  SampleTime=1.0465724751439e-08
  vb : Inport  Port=9  OutDataTypeStr=fixdt(1, 18, 8)  PortDimensions=1  SampleTime=1.0465724751439e-08
  vc : Inport  Port=10  OutDataTypeStr=fixdt(1, 18, 8)  PortDimensions=1  SampleTime=1.0465724751439e-08
  sch_ctr_48 : Inport  Port=11  OutDataTypeStr=fixdt(0, 6, 0)  SampleTime=1.0465724751439e-08
  Data Type Conversion : DataTypeConversion  OutDataTypeStr=fixdt(1, 25, 13)  SampleTime=1.0465724751439e-08  SaturateOnIntegerOverflow=off  RndMeth=Floor
  Data Type Conversion1 : DataTypeConversion  OutDataTypeStr=fixdt(1, 18, 6)  SampleTime=1.0465724751439e-08  SaturateOnIntegerOverflow=off  RndMeth=Floor
  Sparse Matrix-Vector Product : Subsystem
  Sparse Matrix-Vector Product1 : Subsystem
  Sparse Matrix-Vector Product2 : Subsystem
  Sparse Matrix-Vector Product3 : Subsystem
  State : RateTransition  InitialCondition=double(0)  OutPortSampleTimeOpt=Multiple of input port sample time  OutPortSampleTimeMultiple=49
  State_Initial_Val : Constant  Value=[0;0;0;0;0;0;580]  OutDataTypeStr=fixdt(1, 25, 13)  SampleTime=1.0465724751439e-08
  State_absorbed : Delay  DelayLength=0
  State_ctrl_const : Constant  OutDataTypeStr=boolean  SampleTime=5.12820512820513e-07
  State_ctrl_delay : Delay  DelayLength=double(1)  InitialCondition=0  SampleTime=5.12820512820513e-07
  Zero{,1..3} (4 alike) : Constant  Value=0  OutDataTypeStr=boolean  SampleTime=1.0465724751439e-08
  concatenate : Concatenate  NumInputs=10
  crp_out_delay : Delay  DelayLength=double(1)  InitialCondition=0  SampleTime=1.0465724751439e-08
  dtc : hdlmdlgenlib/Buffer
  in0_repeat : RateTransition  Integrity=off  Deterministic=off  OutPortSampleTimeOpt=Multiple of input port sample time  OutPortSampleTimeMultiple=1/49
  in1_repeat : RateTransition  Integrity=off  Deterministic=off  OutPortSampleTimeOpt=Multiple of input port sample time  OutPortSampleTimeMultiple=1/49
  rd_{0..3} (4 alike) : Delay  DelayLength=double(5)  InitialCondition=0  SampleTime=1.0465724751439e-08
  rd_4 : Delay  DelayLength=double(2)  InitialCondition=0  SampleTime=1.0465724751439e-08
  streaming_partition_streamed : Subsystem
  streaming_partition_streamed1 : Subsystem
  sumOuputEqnComp : Sum  OutDataTypeStr=fixdt(1, 25, 13)  SampleTime=1.0465724751439e-08
  t : Demux  Outputs=20
  I_load : Outport  SampleTime=1.0465724751439e-08
  is_out_MOSFET : Outport  Port=2  SampleTime=1.0465724751439e-08
  vs_out_MOSFET : Outport  Port=3  SampleTime=1.0465724751439e-08
  is_out_MOSFET1 : Outport  Port=4  SampleTime=1.0465724751439e-08
  vs_out_MOSFET1 : Outport  Port=5  SampleTime=1.0465724751439e-08
  is_out_MOSFET2 : Outport  Port=6  SampleTime=1.0465724751439e-08
  vs_out_MOSFET2 : Outport  Port=7  SampleTime=1.0465724751439e-08
  is_out_MOSFET3 : Outport  Port=8  SampleTime=1.0465724751439e-08
  vs_out_MOSFET3 : Outport  Port=9  SampleTime=1.0465724751439e-08
  is_out_MOSFET4 : Outport  Port=10  SampleTime=1.0465724751439e-08
  vs_out_MOSFET4 : Outport  Port=11  SampleTime=1.0465724751439e-08
  is_out_MOSFET5 : Outport  Port=12  SampleTime=1.0465724751439e-08
  vs_out_MOSFET5 : Outport  Port=13  SampleTime=1.0465724751439e-08
  Vout : Outport  Port=14  SampleTime=1.0465724751439e-08
  Ib : Outport  Port=15  SampleTime=1.0465724751439e-08
  Ic : Outport  Port=16  SampleTime=1.0465724751439e-08
  Ia : Outport  Port=17  SampleTime=1.0465724751439e-08
  Vb : Outport  Port=18  SampleTime=1.0465724751439e-08
  Vc : Outport  Port=19  SampleTime=1.0465724751439e-08
  Va : Outport  Port=20  SampleTime=1.0465724751439e-08
  wires:
  Sparse Matrix-Vector Product2/1(matrixCOutSignal) -> sumOuputEqnComp/2
  I_load_in/1 -> rd_0/1
  ic_in_MOSFET/1 -> concatenate/2
  vc/1 -> rd_3/1
  va/1 -> rd_1/1
  t/10 -> is_out_MOSFET4/1
  sch_ctr_48/1 -> Sparse Matrix-Vector Product2/3(enb_counter), streaming_partition_streamed/3(enb_counter), Sparse Matrix-Vector Product3/3(enb_counter), Sparse Matrix-Vector Product/3(enb_counter), Sparse Matrix-Vector Product1/3(enb_counter), streaming_partition_streamed1/4(enb_counter)
  vb/1 -> rd_2/1
  t/16 -> Ic/1
  streaming_partition_streamed/1(out0) -> crp_out_delay/1
  ic_in_MOSFET1/1 -> concatenate/3
  ic_in_MOSFET2/1 -> concatenate/4
  Zero1/1 -> Sparse Matrix-Vector Product1/2(selectSignal)
  rd_0/1 -> concatenate/1
  t/15 -> Ib/1
  ic_in_MOSFET3/1 -> concatenate/5
  rd_3/1 -> concatenate/10
  ic_in_MOSFET4/1 -> concatenate/6
  ic_in_MOSFET5/1 -> concatenate/7
  rd_1/1 -> concatenate/8
  rd_2/1 -> concatenate/9
  State_ctrl_const/1 -> State_ctrl_delay/1
  concatenate/1 -> Data Type Conversion/1
  t/11 -> vs_out_MOSFET4/1
  State_ctrl_delay/1 -> in1_repeat/1
  t/18 -> Vb/1
  t/7 -> vs_out_MOSFET2/1
  Zero/1 -> Sparse Matrix-Vector Product/2(selectSignal)
  State/1 -> State_absorbed/1
  Data Type Conversion/1 -> Sparse Matrix-Vector Product3/1(in0), Sparse Matrix-Vector Product/1(in0)
  Sparse Matrix-Vector Product3/1(matrixDOutSignal) -> rd_4/1
  in1_repeat/1 -> streaming_partition_streamed1/2(in1)
  State_Initial_Val/1 -> streaming_partition_streamed1/3(in2)
  Zero3/1 -> Sparse Matrix-Vector Product3/2(selectSignal)
  Sparse Matrix-Vector Product/1(matrixBOutSignal) -> streaming_partition_streamed/1(in0)
  streaming_partition_streamed1/1(out0) -> Sparse Matrix-Vector Product2/1(delayOutSignal), Sparse Matrix-Vector Product1/1(delayOutSignal)
  in0_repeat/1 -> streaming_partition_streamed1/1(in0)
  Zero2/1 -> Sparse Matrix-Vector Product2/2(selectSignal)
  t/2 -> is_out_MOSFET/1
  Sparse Matrix-Vector Product1/1(matrixAOutSignal) -> streaming_partition_streamed/2(in1)
  rd_4/1 -> sumOuputEqnComp/1
  sumOuputEqnComp/1 -> dtc/1
  crp_out_delay/1 -> State/1
  dtc/1 -> Data Type Conversion1/1
  Data Type Conversion1/1 -> t/1
  t/13 -> vs_out_MOSFET5/1
  t/9 -> vs_out_MOSFET3/1
  t/5 -> vs_out_MOSFET1/1
  State_absorbed/1 -> in0_repeat/1
  t/1 -> I_load/1
  t/3 -> vs_out_MOSFET/1
  t/12 -> is_out_MOSFET5/1
  t/4 -> is_out_MOSFET1/1
  t/6 -> is_out_MOSFET2/1
  t/8 -> is_out_MOSFET3/1
  t/14 -> Vout/1
  t/17 -> Ia/1
  t/19 -> Vc/1
  t/20 -> Va/1

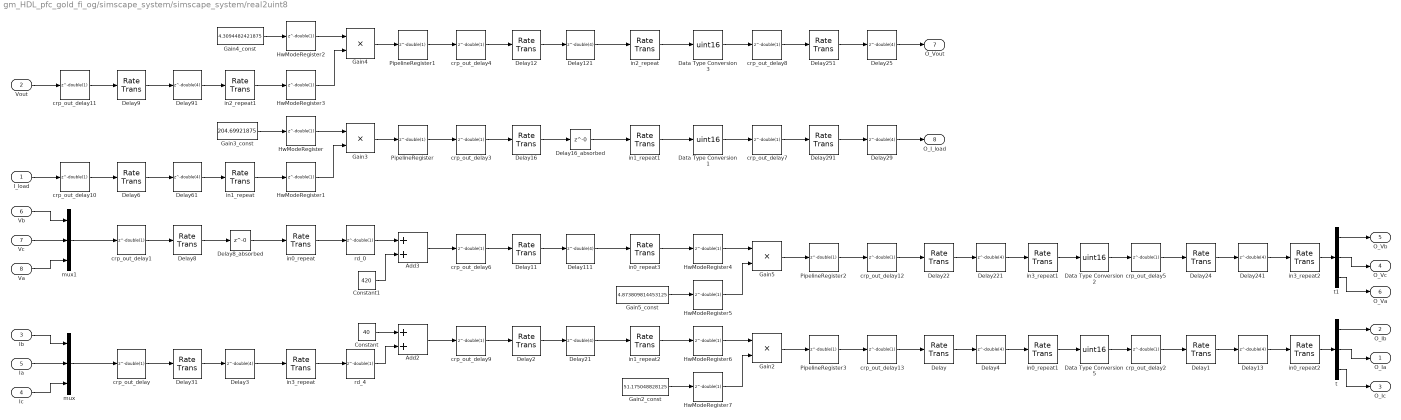
== system gm_HDL_pfc_gold_fi_og/simscape_system/simscape_system/real2uint8 ==
  I_load : Inport  OutDataTypeStr=fixdt(1, 18, 6)  PortDimensions=1  SampleTime=1.0465724751439e-08
  Vout : Inport  Port=2  OutDataTypeStr=fixdt(1, 18, 6)  PortDimensions=1  SampleTime=1.0465724751439e-08
  Ib : Inport  Port=3  OutDataTypeStr=fixdt(1, 18, 6)  PortDimensions=1  SampleTime=1.0465724751439e-08
  Ic : Inport  Port=4  OutDataTypeStr=fixdt(1, 18, 6)  PortDimensions=1  SampleTime=1.0465724751439e-08
  Ia : Inport  Port=5  OutDataTypeStr=fixdt(1, 18, 6)  PortDimensions=1  SampleTime=1.0465724751439e-08
  Vb : Inport  Port=6  OutDataTypeStr=fixdt(1, 18, 6)  PortDimensions=1  SampleTime=1.0465724751439e-08
  Vc : Inport  Port=7  OutDataTypeStr=fixdt(1, 18, 6)  PortDimensions=1  SampleTime=1.0465724751439e-08
  Va : Inport  Port=8  OutDataTypeStr=fixdt(1, 18, 6)  PortDimensions=1  SampleTime=1.0465724751439e-08
  Add2 : Sum  OutDataTypeStr=fixdt(1, 19, 6)  AccumDataTypeStr=fixdt(1, 19, 6)  SampleTime=1.0465724751439e-08
  Add3 : Sum  OutDataTypeStr=fixdt(1, 19, 6)  AccumDataTypeStr=fixdt(1, 19, 6)  SampleTime=1.0465724751439e-08
  Constant : Constant  Value=40  OutDataTypeStr=fixdt(1, 18, 6)  SampleTime=1.0465724751439e-08
  Constant1 : Constant  Value=420  OutDataTypeStr=fixdt(1, 18, 6)  SampleTime=1.0465724751439e-08
  Data Type Conversion{1..3,5} (4 alike) : DataTypeConversion  OutDataTypeStr=uint16  SampleTime=1.0465724751439e-08  SaturateOnIntegerOverflow=off  RndMeth=Floor
  Delay{,1..2,6,8..9,11..12,16,22,24,31,251,291} (14 alike) : RateTransition  InitialCondition=double(0)  OutPortSampleTimeOpt=Multiple of input port sample time  OutPortSampleTimeMultiple=49
  Delay{3..4,13,21,25,29,61,91,111,121,221,241} (12 alike) : Delay  DelayLength=double(4)  InitialCondition=0  SampleTime=5.12820512820513e-07
  Delay16_absorbed : Delay  DelayLength=0
  Delay8_absorbed : Delay  DelayLength=0
  Gain2 : Product  Inputs=**  OutDataTypeStr=fixdt(1, 38, 18)  SampleTime=1.0465724751439e-08
  Gain2_const : Constant  Value=51.175048828125  OutDataTypeStr=fixdt(1, 19, 12)  SampleTime=1.0465724751439e-08
  Gain3 : Product  Inputs=**  OutDataTypeStr=fixdt(1, 36, 15)  SampleTime=1.0465724751439e-08
  Gain3_const : Constant  Value=204.69921875  OutDataTypeStr=fixdt(1, 18, 9)  SampleTime=1.0465724751439e-08
  Gain4 : Product  Inputs=**  OutDataTypeStr=fixdt(1, 36, 20)  SampleTime=1.0465724751439e-08
  Gain4_const : Constant  Value=4.3094482421875  OutDataTypeStr=fixdt(1, 18, 14)  SampleTime=1.0465724751439e-08
  Gain5 : Product  Inputs=**  OutDataTypeStr=fixdt(1, 38, 21)  SampleTime=1.0465724751439e-08
  Gain5_const : Constant  Value=4.873809814453125  OutDataTypeStr=fixdt(1, 19, 15)  SampleTime=1.0465724751439e-08
  HwModeRegister{,1..7} (8 alike) : Delay  DelayLength=double(1)  InitialCondition=0  SampleTime=1.0465724751439e-08
  PipelineRegister{,1..3} (4 alike) : Delay  DelayLength=double(1)  InitialCondition=0  SampleTime=1.0465724751439e-08
  crp_out_delay{,1..13} (14 alike) : Delay  DelayLength=double(1)  InitialCondition=0  SampleTime=1.0465724751439e-08
  in0_repeat{,1..3} (4 alike) : RateTransition  Integrity=off  Deterministic=off  OutPortSampleTimeOpt=Multiple of input port sample time  OutPortSampleTimeMultiple=1/49
  in1_repeat : RateTransition  Integrity=off  Deterministic=off  OutPortSampleTimeOpt=Multiple of input port sample time  OutPortSampleTimeMultiple=1/49
  in1_repeat1 : RateTransition  Integrity=off  Deterministic=off  OutPortSampleTimeOpt=Multiple of input port sample time  OutPortSampleTimeMultiple=1/49
  in1_repeat2 : RateTransition  Integrity=off  Deterministic=off  OutPortSampleTimeOpt=Multiple of input port sample time  OutPortSampleTimeMultiple=1/49
  in2_repeat : RateTransition  Integrity=off  Deterministic=off  OutPortSampleTimeOpt=Multiple of input port sample time  OutPortSampleTimeMultiple=1/49
  in2_repeat1 : RateTransition  Integrity=off  Deterministic=off  OutPortSampleTimeOpt=Multiple of input port sample time  OutPortSampleTimeMultiple=1/49
  in3_repeat : RateTransition  Integrity=off  Deterministic=off  OutPortSampleTimeOpt=Multiple of input port sample time  OutPortSampleTimeMultiple=1/49
  in3_repeat1 : RateTransition  Integrity=off  Deterministic=off  OutPortSampleTimeOpt=Multiple of input port sample time  OutPortSampleTimeMultiple=1/49
  in3_repeat2 : RateTransition  Integrity=off  Deterministic=off  OutPortSampleTimeOpt=Multiple of input port sample time  OutPortSampleTimeMultiple=1/49
  mux : Mux  Inputs=3
  mux1 : Mux  Inputs=3
  rd_0 : Delay  DelayLength=double(1)  InitialCondition=0  SampleTime=1.0465724751439e-08
  rd_4 : Delay  DelayLength=double(1)  InitialCondition=0  SampleTime=1.0465724751439e-08
  t : Demux  Outputs=3
  t1 : Demux  Outputs=3
  O_Ia : Outport  SampleTime=1.0465724751439e-08
  O_Ib : Outport  Port=2  SampleTime=1.0465724751439e-08
  O_Ic : Outport  Port=3  SampleTime=1.0465724751439e-08
  O_Vc : Outport  Port=4  SampleTime=1.0465724751439e-08
  O_Vb : Outport  Port=5  SampleTime=1.0465724751439e-08
  O_Va : Outport  Port=6  SampleTime=1.0465724751439e-08
  O_Vout : Outport  Port=7  SampleTime=5.12820512820513e-07
  O_I_load : Outport  Port=8  SampleTime=5.12820512820513e-07
  wires:
  Delay8_absorbed/1 -> in0_repeat/1
  I_load/1 -> crp_out_delay10/1
  Vout/1 -> crp_out_delay11/1
  Vb/1 -> mux1/1
  crp_out_delay10/1 -> Delay6/1
  Ic/1 -> mux/3
  Vc/1 -> mux1/2
  Delay2/1 -> Delay21/1
  Ia/1 -> mux/2
  Va/1 -> mux1/3
  Delay111/1 -> in0_repeat3/1
  crp_out_delay9/1 -> Delay2/1
  crp_out_delay1/1 -> Delay8/1
  rd_0/1 -> Add3/1
  Ib/1 -> mux/1
  crp_out_delay11/1 -> Delay9/1
  mux1/1 -> crp_out_delay1/1
  mux/1 -> crp_out_delay/1
  Delay9/1 -> Delay91/1
  Delay6/1 -> Delay61/1
  in2_repeat/1 -> Data Type Conversion3/1
  crp_out_delay/1 -> Delay31/1
  PipelineRegister1/1 -> crp_out_delay4/1
  HwModeRegister1/1 -> Gain3/2
  Delay91/1 -> in2_repeat1/1
  Gain3_const/1 -> HwModeRegister/1
  Delay61/1 -> in1_repeat/1
  crp_out_delay6/1 -> Delay11/1
  Delay8/1 -> Delay8_absorbed/1
  Delay31/1 -> Delay3/1
  Gain4_const/1 -> HwModeRegister2/1
  in0_repeat3/1 -> HwModeRegister4/1
  Delay21/1 -> in1_repeat2/1
  in2_repeat1/1 -> HwModeRegister3/1
  Gain3/1 -> PipelineRegister/1
  in0_repeat/1 -> rd_0/1
  in1_repeat/1 -> HwModeRegister1/1
  Add3/1 -> crp_out_delay6/1
  Delay3/1 -> in3_repeat/1
  HwModeRegister2/1 -> Gain4/1
  Add2/1 -> crp_out_delay9/1
  HwModeRegister3/1 -> Gain4/2
  HwModeRegister/1 -> Gain3/1
  in3_repeat/1 -> rd_4/1
  Gain4/1 -> PipelineRegister1/1
  Constant/1 -> Add2/1
  Constant1/1 -> Add3/2
  rd_4/1 -> Add2/2
  PipelineRegister/1 -> crp_out_delay3/1
  crp_out_delay4/1 -> Delay12/1
  Delay16/1 -> Delay16_absorbed/1
  crp_out_delay3/1 -> Delay16/1
  t1/3 -> O_Va/1
  Delay12/1 -> Delay121/1
  Delay121/1 -> in2_repeat/1
  Delay11/1 -> Delay111/1
  HwModeRegister4/1 -> Gain5/1
  Delay16_absorbed/1 -> in1_repeat1/1
  in1_repeat1/1 -> Data Type Conversion1/1
  in1_repeat2/1 -> HwModeRegister6/1
  Gain5_const/1 -> HwModeRegister5/1
  Gain2_const/1 -> HwModeRegister7/1
  Data Type Conversion3/1 -> crp_out_delay8/1
  Data Type Conversion1/1 -> crp_out_delay7/1
  HwModeRegister5/1 -> Gain5/2
  HwModeRegister6/1 -> Gain2/1
  HwModeRegister7/1 -> Gain2/2
  crp_out_delay8/1 -> Delay251/1
  crp_out_delay7/1 -> Delay291/1
  Gain5/1 -> PipelineRegister2/1
  Gain2/1 -> PipelineRegister3/1
  Delay251/1 -> Delay25/1
  Delay291/1 -> Delay29/1
  PipelineRegister2/1 -> crp_out_delay12/1
  PipelineRegister3/1 -> crp_out_delay13/1
  Delay25/1 -> O_Vout/1
  Delay29/1 -> O_I_load/1
  crp_out_delay12/1 -> Delay22/1
  in0_repeat2/1 -> t/1
  crp_out_delay13/1 -> Delay/1
  Delay22/1 -> Delay221/1
  Delay/1 -> Delay4/1
  Delay221/1 -> in3_repeat1/1
  Delay4/1 -> in0_repeat1/1
  in3_repeat1/1 -> Data Type Conversion2/1
  in0_repeat1/1 -> Data Type Conversion5/1
  Data Type Conversion2/1 -> crp_out_delay5/1
  Data Type Conversion5/1 -> crp_out_delay2/1
  crp_out_delay5/1 -> Delay24/1
  crp_out_delay2/1 -> Delay1/1
  Delay24/1 -> Delay241/1
  Delay1/1 -> Delay13/1
  Delay241/1 -> in3_repeat2/1
  Delay13/1 -> in0_repeat2/1
  in3_repeat2/1 -> t1/1
  t1/1 -> O_Vb/1
  t1/2 -> O_Vc/1
  t/1 -> O_Ib/1
  t/2 -> O_Ia/1
  t/3 -> O_Ic/1

== system gm_HDL_pfc_gold_fi_og/Subsystem1/ctrl_pwm/transforms/Claro-Parl Transform ==
  a : Inport
  b : Inport  Port=2
  wt : Inport  Port=3
  Clarke Transform : mcbcontrolslib/Clarke Transform  VariantControl=Variant2  PhaseInput=Two inputs  EnPowerInv=off
  Cos : Trigonometry  Operator=cos
  Park Transform : mcbcontrolslib/Park Transform  PhaseInput=Two inputs  AxisAlignment=D-axis  ThetaInput=Sine and Cosine electrical position  AngleInput=Per-unit  N_points=1024
  Sin : Trigonometry
  d : Outport
  q : Outport  Port=2
  wires:
  Cos/1 -> Park Transform/4
  Sin/1 -> Park Transform/3
  a/1 -> Clarke Transform/1
  wt/1 -> Sin/1, Cos/1
  Clarke Transform/1 -> Park Transform/1  "Valp_sourc"
  Park Transform/1 -> d/1
  Park Transform/2 -> q/1
  b/1 -> Clarke Transform/2
  Clarke Transform/2 -> Park Transform/2  "Vbet_sourc"

== system gm_HDL_pfc_gold_fi_og/Subsystem1/ctrl_pwm/transforms/Claro-Parl Transform1 ==
  a : Inport
  b : Inport  Port=2
  wt : Inport  Port=3
  Clarke Transform : mcbcontrolslib/Clarke Transform  VariantControl=Variant2  PhaseInput=Two inputs  EnPowerInv=off
  Cos : Trigonometry  Operator=cos
  Park Transform : mcbcontrolslib/Park Transform  PhaseInput=Two inputs  AxisAlignment=D-axis  ThetaInput=Sine and Cosine electrical position  AngleInput=Per-unit  N_points=1024
  Sin : Trigonometry
  d : Outport
  q : Outport  Port=2
  wires:
  Cos/1 -> Park Transform/4
  Sin/1 -> Park Transform/3
  a/1 -> Clarke Transform/1
  wt/1 -> Sin/1, Cos/1
  Clarke Transform/1 -> Park Transform/1  "Ialp_sourc"
  Park Transform/1 -> d/1
  Park Transform/2 -> q/1
  b/1 -> Clarke Transform/2
  Clarke Transform/2 -> Park Transform/2  "Ibet_sourc"
